simulink model "cmpy3"  (Simulink 6.2)
settings: Solver=ode45  StartTime=0.0  StopTime=10.0  RelTol=1e-3
values from neighbouring files (symbols this model uses):
  h = 50    [fir_init.m]    (also in r2_dit_fft_init.m; r4_dit_fft_init.m = 80)
libraries: xbsIndex_r3 x57
settings Model: LastModifiedBy=mdexter
settings DebuggingCC: SolverPrmCheckMsg=warning

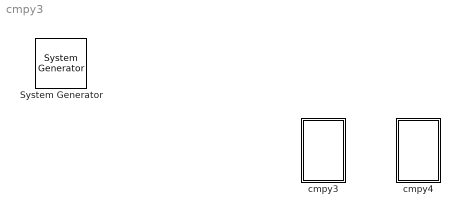
== system cmpy3 ==
  " System Generator" : xbsIndex_r3/ System Generator  Tag=genX  xilinxfamily=Virtex2  part=xc2v1000  speed=-4  package=bg575  synthesis_tool=XST  directory=./netlist  testbench=off  simulink_period=1  sysclk_period=100  incr_netlist=off  trim_vbits=Everywhere in SubSystem  dbl_ovrd=According to Block Masks  core_generation=According to Block Masks  run_coregen=off  deprecated_control=off  eval_field=0
      settings: AttributesFormatString=System\nGenerator
  cmpy3 : Subsystem
  cmpy4 : Subsystem

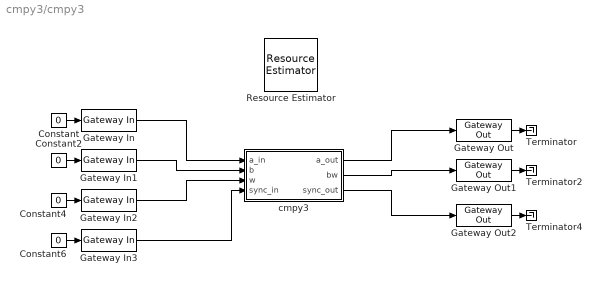
== system cmpy3/cmpy3 ==
  Constant{,2,4,6} (4 alike) : Constant  Value=0
  Gateway In : xbsIndex_r3/Gateway In  arith_type=Unsigned  n_bits=34  bin_pt=0  quantization=Truncate  overflow=Wrap  period=1  timing_constraint=None  locs_specified=off  LOCs={}  needs_fixed_name=off  dbl_ovrd=off  show_param=off
      settings: xl_area=[0 0 0 0 34 0 0]
  Gateway In1 : xbsIndex_r3/Gateway In  arith_type=Unsigned  n_bits=34  bin_pt=0  quantization=Truncate  overflow=Wrap  period=1  timing_constraint=None  locs_specified=off  LOCs={}  needs_fixed_name=off  dbl_ovrd=off  show_param=off
      settings: xl_area=[0 0 0 0 34 0 0]
  Gateway In2 : xbsIndex_r3/Gateway In  arith_type=Unsigned  n_bits=18  bin_pt=0  quantization=Truncate  overflow=Wrap  period=1  timing_constraint=None  locs_specified=off  LOCs={}  needs_fixed_name=off  dbl_ovrd=off  show_param=off
      settings: xl_area=[0 0 0 0 18 0 0]
  Gateway In3 : xbsIndex_r3/Gateway In  arith_type=Boolean  n_bits=8  bin_pt=6  quantization=Truncate  overflow=Wrap  period=1  timing_constraint=None  locs_specified=off  LOCs={}  needs_fixed_name=off  dbl_ovrd=off  show_param=off
      settings: xl_area=[0 0 0 0 1 0 0]
  Gateway Out : xbsIndex_r3/Gateway Out  output_type=Double  nbits=8  bin_pt=6  arith_type=Boolean  quantization=Truncate  overflow=Wrap  hdl_port=on  timing_constraint=None  locs_specified=off  LOCs={}  needs_fixed_name=off  show_param=off
      settings: xl_area=[0 0 0 0 34 0 0]
  Gateway Out1 : xbsIndex_r3/Gateway Out  output_type=Double  nbits=8  bin_pt=6  arith_type=Boolean  quantization=Truncate  overflow=Wrap  hdl_port=on  timing_constraint=None  locs_specified=off  LOCs={}  needs_fixed_name=off  show_param=off
      settings: xl_area=[0 0 0 0 34 0 0]
  Gateway Out2 : xbsIndex_r3/Gateway Out  output_type=Double  nbits=8  bin_pt=6  arith_type=Boolean  quantization=Truncate  overflow=Wrap  hdl_port=on  timing_constraint=None  locs_specified=off  LOCs={}  needs_fixed_name=off  show_param=off
      settings: xl_area=[0 0 0 0 1 0 0]
  Resource Estimator : xbsIndex_r3/Resource Estimator  Tag=resEstTag  xl_estimator_area=[216 323 0 329 156 3 0]  xl_use_estimator_area=off  simulink_period=1  mrp_directory=h:\dev\newfft.fun
      settings: AttributesFormatString=Resource Estimator\n%<xl_estimator_area>\n[SL FF BR LUT IO MUL TBUF]
  Terminator : Terminator
  Terminator2 : Terminator
  Terminator4 : Terminator
  cmpy3 : Subsystem  mask(Complex Multiplier (4 real multipliers)){n_bits_b=8, bin_pt_b=7, n_bits_w=9, bin_pt_w=7, n_bits_bw=8, bin_pt_bw=7, quantization=Round  (unbiased: +/- Inf), overflow=Saturate, mult_latency=3, add_latency=1}
      mask prompts: n_bits_b "Number of Bits B"; bin_pt_b "Binary Point B"; n_bits_w "Number of Bits W"; bin_pt_w "Binary Point W"; n_bits_bw "Number of Bits BW"; bin_pt_bw "Binary Point BW"; mult_latency "Multiplier Latency"; add_latency "Adder Latency"
      mask help: This block multiplies two complex numbers using 4 real multipliers and 2 real adders. Pass-through paths are provided for another complex number and a sync signal. These pass through paths provide delay that matches the latency of the complex multiply operation.
      mask init:
      | cmpy3_init(gcb, ...
      |     n_bits_b,bin_pt_b, ...
      |     n_bits_w,bin_pt_w, ...
      |     n_bits_bw,bin_pt_bw, ...
      |     quantization,overflow, ...
      |     mult_latency,add_latency);
      settings: AttributesFormatString=8_7 * 9_7 ==> 8_7
      mask Help:
      | <pre>
      | Description::
      | 
      | This block multiplies two complex numbers using 4 real multipliers and 2 real adders.
      | Pass-through paths are provided for another complex number and a sync signal.
      | These paths provide delay that matches the latency of the complex multiply operation.
      | 
      | a_in is passed through to a_out.
      | b and w complex inputs are multiplied and their product appears on the bw output.
      | sync_in is passed through to sync_out.
      | 
      | Mask Parameters::
      | 
      | Number of Bits B (n_bits_b): Specifies the width of the real/imaginary
      | components of input b.  Assumed equal for both components.
      | 
      | Binary Point B (bin_pt_b): Specifies the binary point point position of the
      | real/imaginary components of input b.  Assumed equal for both components.
      | 
      | Number of Bits W (n_bits_w): Specifies the width of the real/imaginary
      | components of input w.  Assumed equal for both components.
      | 
      | Binary Point W (bin_pt_w): Specifies the binary point point position of the
      | real/imaginary components of input w.  Assumed equal for both components.
      | 
      | Number of Bits BW (n_bits_bw): Specifies the width of the real/imaginary
      | components of output bw.  Assumed equal for both components.
      | 
      | Binary Point BW (bin_pt_bw): Specifies the binary point point position of the
      | real/imaginary components of output bw.  Assumed equal for both components.
      | 
      | Quantization (quantization): Specifies quantization handling.
      | 
      | Overflow (overflow): Specifies overflow handling.
      | 
      | Multiplier Latency (mult_latency): Latency to use for the underlying real multipliers.
      | 
      | Adder Latency (add_latency): Latency to use for the underlying real adders.
      | </pre>
      mask StyleString: edit,edit,edit,edit,edit,edit,popup(Truncate|Round  (unbiased: +/- Inf)),popup(Wrap|Saturate|Error),edit,edit
  wires:
  Gateway In/1 -> cmpy3/1(a_in)
  cmpy3/1(a_out) -> Gateway Out/1
  Gateway In1/1 -> cmpy3/2(b)
  cmpy3/2(bw) -> Gateway Out1/1
  Gateway In2/1 -> cmpy3/3(w)
  cmpy3/3(sync_out) -> Gateway Out2/1
  Gateway In3/1 -> cmpy3/4(sync_in)
  Constant/1 -> Gateway In/1
  Constant2/1 -> Gateway In1/1
  Constant4/1 -> Gateway In2/1
  Constant6/1 -> Gateway In3/1
  Gateway Out/1 -> Terminator/1
  Gateway Out1/1 -> Terminator2/1
  Gateway Out2/1 -> Terminator4/1

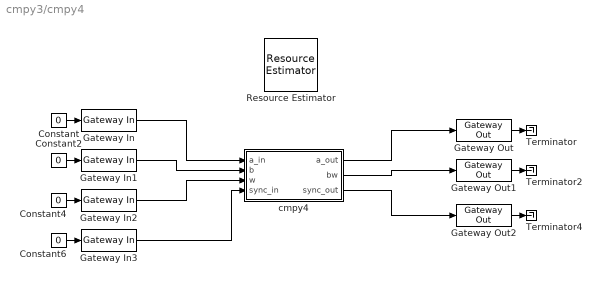
== system cmpy3/cmpy4 ==
  Constant{,2,4,6} (4 alike) : Constant  Value=0
  Gateway In : xbsIndex_r3/Gateway In  arith_type=Unsigned  n_bits=34  bin_pt=0  quantization=Truncate  overflow=Wrap  period=1  timing_constraint=None  locs_specified=off  LOCs={}  needs_fixed_name=off  dbl_ovrd=off  show_param=off
      settings: xl_area=[0 0 0 0 34 0 0]
  Gateway In1 : xbsIndex_r3/Gateway In  arith_type=Unsigned  n_bits=34  bin_pt=0  quantization=Truncate  overflow=Wrap  period=1  timing_constraint=None  locs_specified=off  LOCs={}  needs_fixed_name=off  dbl_ovrd=off  show_param=off
      settings: xl_area=[0 0 0 0 34 0 0]
  Gateway In2 : xbsIndex_r3/Gateway In  arith_type=Unsigned  n_bits=18  bin_pt=0  quantization=Truncate  overflow=Wrap  period=1  timing_constraint=None  locs_specified=off  LOCs={}  needs_fixed_name=off  dbl_ovrd=off  show_param=off
      settings: xl_area=[0 0 0 0 18 0 0]
  Gateway In3 : xbsIndex_r3/Gateway In  arith_type=Boolean  n_bits=8  bin_pt=6  quantization=Truncate  overflow=Wrap  period=1  timing_constraint=None  locs_specified=off  LOCs={}  needs_fixed_name=off  dbl_ovrd=off  show_param=off
      settings: xl_area=[0 0 0 0 1 0 0]
  Gateway Out : xbsIndex_r3/Gateway Out  output_type=Double  nbits=8  bin_pt=6  arith_type=Boolean  quantization=Truncate  overflow=Wrap  hdl_port=on  timing_constraint=None  locs_specified=off  LOCs={}  needs_fixed_name=off  show_param=off
      settings: xl_area=[0 0 0 0 34 0 0]
  Gateway Out1 : xbsIndex_r3/Gateway Out  output_type=Double  nbits=8  bin_pt=6  arith_type=Boolean  quantization=Truncate  overflow=Wrap  hdl_port=on  timing_constraint=None  locs_specified=off  LOCs={}  needs_fixed_name=off  show_param=off
      settings: xl_area=[0 0 0 0 34 0 0]
  Gateway Out2 : xbsIndex_r3/Gateway Out  output_type=Double  nbits=8  bin_pt=6  arith_type=Boolean  quantization=Truncate  overflow=Wrap  hdl_port=on  timing_constraint=None  locs_specified=off  LOCs={}  needs_fixed_name=off  show_param=off
      settings: xl_area=[0 0 0 0 1 0 0]
  Resource Estimator : xbsIndex_r3/Resource Estimator  Tag=resEstTag  xl_estimator_area=[210 297 0 311 156 4 0]  xl_use_estimator_area=off  simulink_period=1  mrp_directory=h:\dev\newfft.fun
      settings: AttributesFormatString=Resource Estimator\n%<xl_estimator_area>\n[SL FF BR LUT IO MUL TBUF]
  Terminator : Terminator
  Terminator2 : Terminator
  Terminator4 : Terminator
  cmpy4 : Subsystem  mask(Complex Multiplier (4 real multipliers)){n_bits_b=17, bin_pt_b=7, n_bits_w=9, bin_pt_w=7, n_bits_bw=17, bin_pt_bw=7, quantization=Round  (unbiased: +/- Inf), overflow=Saturate, mult_latency=3, add_latency=1}
      mask prompts: n_bits_b "Number of Bits B"; bin_pt_b "Binary Point B"; n_bits_w "Number of Bits W"; bin_pt_w "Binary Point W"; n_bits_bw "Number of Bits BW"; bin_pt_bw "Binary Point BW"; mult_latency "Multiplier Latency"; add_latency "Adder Latency"
      mask help: This block multiplies two complex numbers using 4 real multipliers and 2 real adders. Pass-through paths are provided for another complex number and a sync signal. These pass through paths provide delay that matches the latency of the complex multiply operation.
      mask init:
      | cmpy4_init(gcb, ...
      |     n_bits_b,bin_pt_b, ...
      |     n_bits_w,bin_pt_w, ...
      |     n_bits_bw,bin_pt_bw, ...
      |     quantization,overflow, ...
      |     mult_latency,add_latency);
      settings: AttributesFormatString=17_7 * 9_7 ==> 17_7
      mask Help:
      | <pre>
      | Description::
      | 
      | This block multiplies two complex numbers using 4 real multipliers and 2 real adders.
      | Pass-through paths are provided for another complex number and a sync signal.
      | These paths provide delay that matches the latency of the complex multiply operation.
      | 
      | a_in is passed through to a_out.
      | b and w complex inputs are multiplied and their product appears on the bw output.
      | sync_in is passed through to sync_out.
      | 
      | Mask Parameters::
      | 
      | Number of Bits B (n_bits_b): Specifies the width of the real/imaginary
      | components of input b.  Assumed equal for both components.
      | 
      | Binary Point B (bin_pt_b): Specifies the binary point point position of the
      | real/imaginary components of input b.  Assumed equal for both components.
      | 
      | Number of Bits W (n_bits_w): Specifies the width of the real/imaginary
      | components of input w.  Assumed equal for both components.
      | 
      | Binary Point W (bin_pt_w): Specifies the binary point point position of the
      | real/imaginary components of input w.  Assumed equal for both components.
      | 
      | Number of Bits BW (n_bits_bw): Specifies the width of the real/imaginary
      | components of output bw.  Assumed equal for both components.
      | 
      | Binary Point BW (bin_pt_bw): Specifies the binary point point position of the
      | real/imaginary components of output bw.  Assumed equal for both components.
      | 
      | Quantization (quantization): Specifies quantization handling.
      | 
      | Overflow (overflow): Specifies overflow handling.
      | 
      | Multiplier Latency (mult_latency): Latency to use for the underlying real multipliers.
      | 
      | Adder Latency (add_latency): Latency to use for the underlying real adders.
      | </pre>
      mask StyleString: edit,edit,edit,edit,edit,edit,popup(Truncate|Round  (unbiased: +/- Inf)),popup(Wrap|Saturate|Error),edit,edit
  wires:
  Gateway In/1 -> cmpy4/1(a_in)
  cmpy4/1(a_out) -> Gateway Out/1
  Gateway In1/1 -> cmpy4/2(b)
  cmpy4/2(bw) -> Gateway Out1/1
  Gateway In2/1 -> cmpy4/3(w)
  cmpy4/3(sync_out) -> Gateway Out2/1
  Gateway In3/1 -> cmpy4/4(sync_in)
  Constant/1 -> Gateway In/1
  Constant2/1 -> Gateway In1/1
  Constant4/1 -> Gateway In2/1
  Constant6/1 -> Gateway In3/1
  Gateway Out/1 -> Terminator/1
  Gateway Out1/1 -> Terminator2/1
  Gateway Out2/1 -> Terminator4/1

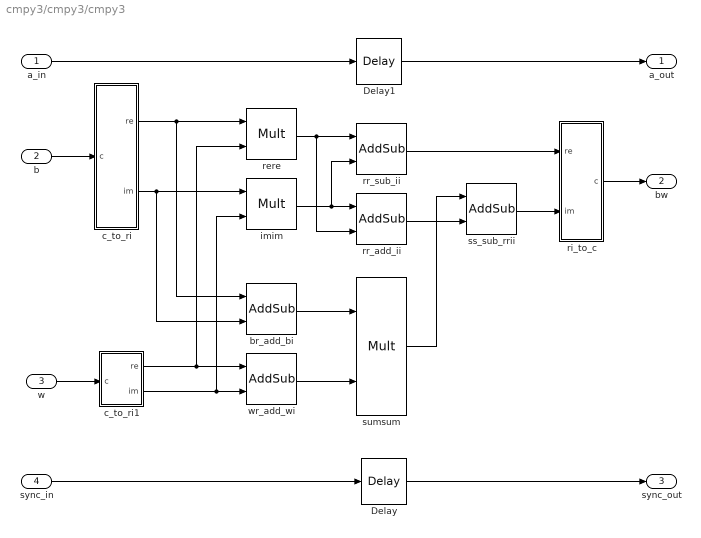
== system cmpy3/cmpy3/cmpy3 ==
  a_in : Inport  Port=1  LatchInput=off
  b : Inport  Port=2  LatchInput=off
  w : Inport  Port=3  LatchInput=off
  sync_in : Inport  Port=4  LatchInput=off
  Delay : xbsIndex_r3/Delay  latency=5  reg_retiming=off  explicit_period=off  period=1  en=off  accept_only_valid=off  init_zero=on  dbl_ovrd=off  show_param=off
      settings: xl_area=[1 1 0 1 0 0 0]
  Delay1 : xbsIndex_r3/Delay  latency=5  reg_retiming=off  explicit_period=off  period=1  en=off  accept_only_valid=off  init_zero=on  dbl_ovrd=off  show_param=off
      settings: xl_area=[17 34 0 34 0 0 0]
  br_add_bi : xbsIndex_r3/AddSub  mode=Addition  precision=Full  arith_type=Unsigned  n_bits=8  bin_pt=2  quantization=Truncate  overflow=Wrap  latency=1  explicit_period=off  period=1  use_carryin=off  use_carryout=off  en=off  dbl_ovrd=off  show_param=on  use_core=on  pipeline=on  use_rpm=on  gen_core=off
      settings: xl_area=[9 18 0 18 0 0 0]
  c_to_ri : Subsystem  mask(Complex to Real-Imag){n_bits=8, bin_pt=7}
      mask prompts: n_bits "Bit Width"; bin_pt "Binary Point"
      mask help: Outputs real and imaginary components of a complex input.
      settings: AttributesFormatString=8_7 r/i
      mask Help:
      | <pre>
      | Description::
      | 
      | Outputs real and imaginary components of a complex input.
      | Useful for simplifying interconnects.
      | See also: Real-Imag to Complex (ri_to_c)
      | 
      | Mask Parameters::
      | 
      | Bit Width (n_bits): Specifies the width of the real/imaginary components.
      | Assumed equal for both components.
      | 
      | Binary Point (bin_pt): Specifies the binary point location in the real/imaginary components.
      | Assumed equal for both components.
      | </pre>
  c_to_ri1 : Subsystem  mask(Complex to Real-Imag){n_bits=9, bin_pt=7}
      mask prompts: n_bits "Bit Width"; bin_pt "Binary Point"
      mask help: Outputs real and imaginary components of a complex input.
      mask init:
      | c_to_ri_init(gcb,n_bits,bin_pt);
      settings: AttributesFormatString=9_7 r/i
      mask Help:
      | <pre>
      | Description::
      | 
      | Outputs real and imaginary components of a complex input.
      | Useful for simplifying interconnects.
      | See also: Real-Imag to Complex (ri_to_c)
      | 
      | Mask Parameters::
      | 
      | Bit Width (n_bits): Specifies the width of the real/imaginary components.
      | Assumed equal for both components.
      | 
      | Binary Point (bin_pt): Specifies the binary point location in the real/imaginary components.
      | Assumed equal for both components.
      | </pre>
  imim : xbsIndex_r3/Mult  precision=Full  arith_type="Signed  (2's comp)"  n_bits=8  bin_pt=2  quantization=Truncate  overflow=Wrap  latency=3  explicit_period=off  period=1  en=off  dbl_ovrd=off  show_param=on  mult_type=Parallel  oversample=2  use_embedded=on  pipeline=on  use_rpm=on  placement_style=Rectangular Shape  gen_core=off
      settings: xl_area=[26 52 0 26 0 1 0]
  rere : xbsIndex_r3/Mult  precision=Full  arith_type="Signed  (2's comp)"  n_bits=8  bin_pt=2  quantization=Truncate  overflow=Wrap  latency=3  explicit_period=off  period=1  en=off  dbl_ovrd=off  show_param=on  mult_type=Parallel  oversample=2  use_embedded=on  pipeline=on  use_rpm=on  placement_style=Rectangular Shape  gen_core=off
      settings: xl_area=[26 52 0 26 0 1 0]
  ri_to_c : Subsystem  mask(Real-Imag to Complex){}
      mask help: Concatenates real and imaginary inputs into a complex output.
      mask init:
      | ri_to_c_init(gcb);
      mask Help:
      | <pre>
      | Description::
      | 
      | Concatenates a real and imaginary input into a complex output.
      | Useful for simplifying interconnects.
      | See also: Complex to Real-Imag (c_to_ri)
      | 
      | Mask Parameters::
      | 
      | (N/A)
      | </pre>
  rr_add_ii : xbsIndex_r3/AddSub  mode=Addition  precision=Full  arith_type=Unsigned  n_bits=8  bin_pt=2  quantization=Truncate  overflow=Wrap  latency=1  explicit_period=off  period=1  use_carryin=off  use_carryout=off  en=off  dbl_ovrd=off  show_param=on  use_core=on  pipeline=on  use_rpm=on  gen_core=off
      settings: xl_area=[14 27 0 27 0 0 0]
  rr_sub_ii : xbsIndex_r3/AddSub  mode=Subtraction  precision=User Defined  arith_type=Unsigned  n_bits=8  bin_pt=7  quantization="Round  (unbiased: +/- Inf)"  overflow=Saturate  latency=2  explicit_period=off  period=1  use_carryin=off  use_carryout=off  en=off  dbl_ovrd=off  show_param=on  use_core=on  pipeline=on  use_rpm=on  gen_core=off
      settings: xl_area=[44 44 0 69 0 0 0]
  ss_sub_rrii : xbsIndex_r3/AddSub  mode=Subtraction  precision=User Defined  arith_type="Signed  (2's comp)"  n_bits=8  bin_pt=7  quantization="Round  (unbiased: +/- Inf)"  overflow=Saturate  latency=1  explicit_period=off  period=1  use_carryin=off  use_carryout=off  en=off  dbl_ovrd=off  show_param=on  use_core=on  pipeline=on  use_rpm=on  gen_core=off
      settings: xl_area=[46 29 0 90 0 0 0]
  sumsum : xbsIndex_r3/Mult  precision=Full  arith_type="Signed  (2's comp)"  n_bits=8  bin_pt=2  quantization=Truncate  overflow=Wrap  latency=3  explicit_period=off  period=1  en=off  dbl_ovrd=off  show_param=on  mult_type=Parallel  oversample=2  use_embedded=on  pipeline=on  use_rpm=on  placement_style=Rectangular Shape  gen_core=off
      settings: xl_area=[28 56 0 28 0 1 0]
  wr_add_wi : xbsIndex_r3/AddSub  mode=Addition  precision=Full  arith_type=Unsigned  n_bits=8  bin_pt=2  quantization=Truncate  overflow=Wrap  latency=1  explicit_period=off  period=1  use_carryin=off  use_carryout=off  en=off  dbl_ovrd=off  show_param=on  use_core=on  pipeline=on  use_rpm=on  gen_core=off
      settings: xl_area=[5 10 0 10 0 0 0]
  a_out : Outport
  bw : Outport  Port=2
  sync_out : Outport  Port=3
  wires:
  Delay1/1 -> a_out/1
  a_in/1 -> Delay1/1
  c_to_ri/2(im) -> imim/1, br_add_bi/2
  c_to_ri1/1(re) -> wr_add_wi/1, rere/2
  c_to_ri1/2(im) -> wr_add_wi/2, imim/2
  c_to_ri/1(re) -> rere/1, br_add_bi/1
  Delay/1 -> sync_out/1
  sync_in/1 -> Delay/1
  sumsum/1 -> ss_sub_rrii/1
  ri_to_c/1(c) -> bw/1
  wr_add_wi/1 -> sumsum/2
  br_add_bi/1 -> sumsum/1
  imim/1 -> rr_add_ii/1, rr_sub_ii/2
  rere/1 -> rr_sub_ii/1, rr_add_ii/2
  w/1 -> c_to_ri1/1(c)
  b/1 -> c_to_ri/1(c)
  rr_add_ii/1 -> ss_sub_rrii/2
  rr_sub_ii/1 -> ri_to_c/1(re)
  ss_sub_rrii/1 -> ri_to_c/2(im)

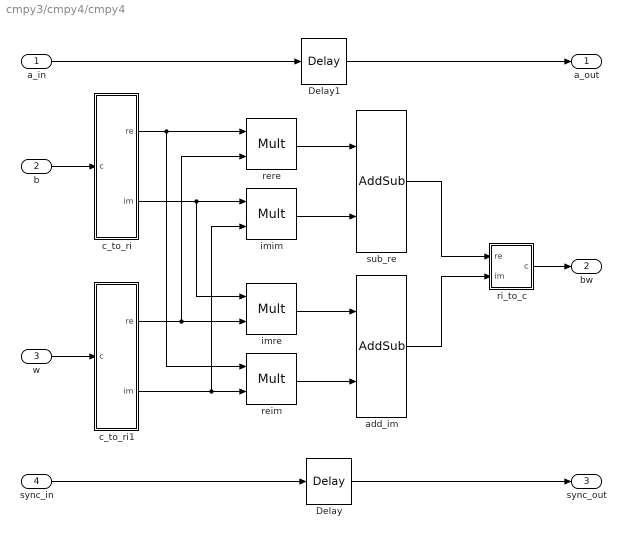
== system cmpy3/cmpy4/cmpy4 ==
  a_in : Inport  Port=1  LatchInput=off
  b : Inport  Port=2  LatchInput=off
  w : Inport  Port=3  LatchInput=off
  sync_in : Inport  Port=4  LatchInput=off
  Delay : xbsIndex_r3/Delay  latency=4  reg_retiming=off  explicit_period=off  period=1  en=off  accept_only_valid=off  init_zero=on  dbl_ovrd=off  show_param=off
      settings: xl_area=[1 1 0 1 0 0 0]
  Delay1 : xbsIndex_r3/Delay  latency=4  reg_retiming=off  explicit_period=off  period=1  en=off  accept_only_valid=off  init_zero=on  dbl_ovrd=off  show_param=off
      settings: xl_area=[17 34 0 34 0 0 0]
  add_im : xbsIndex_r3/AddSub  mode=Addition  precision=User Defined  arith_type="Signed  (2's comp)"  n_bits=17  bin_pt=7  quantization="Round  (unbiased: +/- Inf)"  overflow=Saturate  latency=1  explicit_period=off  period=1  use_carryin=off  use_carryout=off  en=off  dbl_ovrd=off  show_param=on  use_core=on  pipeline=on  use_rpm=on  gen_core=off
      settings: xl_area=[44 27 0 86 0 0 0]
  c_to_ri : Subsystem  mask(Complex to Real-Imag){n_bits=17, bin_pt=7}
      mask prompts: n_bits "Bit Width"; bin_pt "Binary Point"
      mask help: Outputs real and imaginary components of a complex input.
      settings: AttributesFormatString=17_7 r/i
      mask Help:
      | <pre>
      | Description::
      | 
      | Outputs real and imaginary components of a complex input.
      | Useful for simplifying interconnects.
      | See also: Real-Imag to Complex (ri_to_c)
      | 
      | Mask Parameters::
      | 
      | Bit Width (n_bits): Specifies the width of the real/imaginary components.
      | Assumed equal for both components.
      | 
      | Binary Point (bin_pt): Specifies the binary point location in the real/imaginary components.
      | Assumed equal for both components.
      | </pre>
  c_to_ri1 : Subsystem  mask(Complex to Real-Imag){n_bits=9, bin_pt=7}
      mask prompts: n_bits "Bit Width"; bin_pt "Binary Point"
      mask help: Outputs real and imaginary components of a complex input.
      settings: AttributesFormatString=9_7 r/i
      mask Help:
      | <pre>
      | Description::
      | 
      | Outputs real and imaginary components of a complex input.
      | Useful for simplifying interconnects.
      | See also: Real-Imag to Complex (ri_to_c)
      | 
      | Mask Parameters::
      | 
      | Bit Width (n_bits): Specifies the width of the real/imaginary components.
      | Assumed equal for both components.
      | 
      | Binary Point (bin_pt): Specifies the binary point location in the real/imaginary components.
      | Assumed equal for both components.
      | </pre>
  imim : xbsIndex_r3/Mult  precision=Full  arith_type="Signed  (2's comp)"  n_bits=8  bin_pt=2  quantization=Truncate  overflow=Wrap  latency=3  explicit_period=off  period=1  en=off  dbl_ovrd=off  show_param=on  mult_type=Parallel  oversample=2  use_embedded=on  pipeline=on  use_rpm=on  placement_style=Rectangular Shape  gen_core=off
      settings: xl_area=[26 52 0 26 0 1 0]
  imre : xbsIndex_r3/Mult  precision=Full  arith_type="Signed  (2's comp)"  n_bits=8  bin_pt=2  quantization=Truncate  overflow=Wrap  latency=3  explicit_period=off  period=1  en=off  dbl_ovrd=off  show_param=on  mult_type=Parallel  oversample=2  use_embedded=on  pipeline=on  use_rpm=on  placement_style=Rectangular Shape  gen_core=off
      settings: xl_area=[26 52 0 26 0 1 0]
  reim : xbsIndex_r3/Mult  precision=Full  arith_type="Signed  (2's comp)"  n_bits=8  bin_pt=2  quantization=Truncate  overflow=Wrap  latency=3  explicit_period=off  period=1  en=off  dbl_ovrd=off  show_param=on  mult_type=Parallel  oversample=2  use_embedded=on  pipeline=on  use_rpm=on  placement_style=Rectangular Shape  gen_core=off
      settings: xl_area=[26 52 0 26 0 1 0]
  rere : xbsIndex_r3/Mult  precision=Full  arith_type="Signed  (2's comp)"  n_bits=8  bin_pt=2  quantization=Truncate  overflow=Wrap  latency=3  explicit_period=off  period=1  en=off  dbl_ovrd=off  show_param=on  mult_type=Parallel  oversample=2  use_embedded=on  pipeline=on  use_rpm=on  placement_style=Rectangular Shape  gen_core=off
      settings: xl_area=[26 52 0 26 0 1 0]
  ri_to_c : Subsystem  mask(Real-Imag to Complex){}
      mask help: Concatenates real and imaginary inputs into a complex output.
      mask init:
      | ri_to_c_init(gcb);
      mask Help:
      | <pre>
      | Description::
      | 
      | Concatenates a real and imaginary input into a complex output.
      | Useful for simplifying interconnects.
      | See also: Complex to Real-Imag (c_to_ri)
      | 
      | Mask Parameters::
      | 
      | (N/A)
      | </pre>
  sub_re : xbsIndex_r3/AddSub  mode=Subtraction  precision=User Defined  arith_type="Signed  (2's comp)"  n_bits=17  bin_pt=7  quantization="Round  (unbiased: +/- Inf)"  overflow=Saturate  latency=1  explicit_period=off  period=1  use_carryin=off  use_carryout=off  en=off  dbl_ovrd=off  show_param=on  use_core=on  pipeline=on  use_rpm=on  gen_core=off
      settings: xl_area=[44 27 0 86 0 0 0]
  a_out : Outport
  bw : Outport  Port=2
  sync_out : Outport  Port=3
  wires:
  Delay1/1 -> a_out/1
  a_in/1 -> Delay1/1
  c_to_ri/2(im) -> imre/1, imim/1
  c_to_ri1/1(re) -> rere/2, imre/2
  c_to_ri1/2(im) -> imim/2, reim/2
  c_to_ri/1(re) -> reim/1, rere/1
  Delay/1 -> sync_out/1
  sync_in/1 -> Delay/1
  add_im/1 -> ri_to_c/2(im)
  ri_to_c/1(c) -> bw/1
  sub_re/1 -> ri_to_c/1(re)
  reim/1 -> add_im/2
  imre/1 -> add_im/1
  imim/1 -> sub_re/2
  rere/1 -> sub_re/1
  w/1 -> c_to_ri1/1(c)
  b/1 -> c_to_ri/1(c)

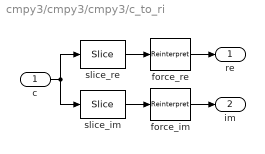
== system cmpy3/cmpy3/cmpy3/c_to_ri ==
  c : Inport  Port=1  LatchInput=off
  force_im : xbsIndex_r3/Reinterpret  force_arith_type=on  arith_type="Signed  (2's comp)"  force_bin_pt=on  bin_pt=7  force_valid=on
  force_re : xbsIndex_r3/Reinterpret  force_arith_type=on  arith_type="Signed  (2's comp)"  force_bin_pt=on  bin_pt=7  force_valid=on
  slice_im : xbsIndex_r3/Slice  mode=Lower Bit Location + Width  nbits=8  bit1=0  base1=MSB of Input  bit0=0  base0=LSB of Input  boolean_output=off  explicit_period=off  period=1  dbl_ovrd=off
  slice_re : xbsIndex_r3/Slice  mode=Upper Bit Location + Width  nbits=8  bit1=0  base1=MSB of Input  bit0=0  base0=LSB of Input  boolean_output=off  explicit_period=off  period=1  dbl_ovrd=off
  re : Outport
  im : Outport  Port=2
  wires:
  slice_re/1 -> force_re/1
  slice_im/1 -> force_im/1
  force_re/1 -> re/1
  force_im/1 -> im/1
  c/1 -> slice_re/1, slice_im/1

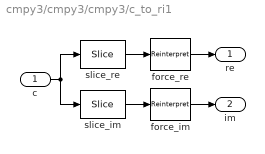
== system cmpy3/cmpy3/cmpy3/c_to_ri1 ==
  c : Inport  Port=1  LatchInput=off
  force_im : xbsIndex_r3/Reinterpret  force_arith_type=on  arith_type="Signed  (2's comp)"  force_bin_pt=on  bin_pt=7  force_valid=on
  force_re : xbsIndex_r3/Reinterpret  force_arith_type=on  arith_type="Signed  (2's comp)"  force_bin_pt=on  bin_pt=7  force_valid=on
  slice_im : xbsIndex_r3/Slice  mode=Lower Bit Location + Width  nbits=9  bit1=0  base1=MSB of Input  bit0=0  base0=LSB of Input  boolean_output=off  explicit_period=off  period=1  dbl_ovrd=off
  slice_re : xbsIndex_r3/Slice  mode=Upper Bit Location + Width  nbits=9  bit1=0  base1=MSB of Input  bit0=0  base0=LSB of Input  boolean_output=off  explicit_period=off  period=1  dbl_ovrd=off
  re : Outport
  im : Outport  Port=2
  wires:
  c/1 -> slice_im/1, slice_re/1
  force_im/1 -> im/1
  force_re/1 -> re/1
  slice_im/1 -> force_im/1
  slice_re/1 -> force_re/1

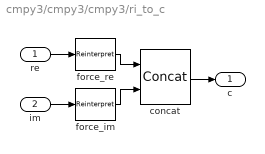
== system cmpy3/cmpy3/cmpy3/ri_to_c ==
  re : Inport  Port=1  LatchInput=off
  im : Inport  Port=2  LatchInput=off
  concat : xbsIndex_r3/Concat  num_inputs=2  explicit_period=off  period=1  dbl_ovrd=off
  force_im : xbsIndex_r3/Reinterpret  force_arith_type=on  arith_type=Unsigned  force_bin_pt=on  bin_pt=0  force_valid=on
  force_re : xbsIndex_r3/Reinterpret  force_arith_type=on  arith_type=Unsigned  force_bin_pt=on  bin_pt=0  force_valid=on
  c : Outport
  wires:
  im/1 -> force_im/1
  concat/1 -> c/1
  re/1 -> force_re/1
  force_im/1 -> concat/2
  force_re/1 -> concat/1

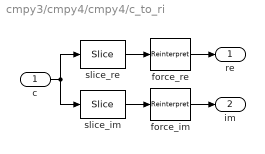
== system cmpy3/cmpy4/cmpy4/c_to_ri ==
  c : Inport  Port=1  LatchInput=off
  force_im : xbsIndex_r3/Reinterpret  force_arith_type=on  arith_type="Signed  (2's comp)"  force_bin_pt=on  bin_pt=7  force_valid=on
  force_re : xbsIndex_r3/Reinterpret  force_arith_type=on  arith_type="Signed  (2's comp)"  force_bin_pt=on  bin_pt=7  force_valid=on
  slice_im : xbsIndex_r3/Slice  mode=Lower Bit Location + Width  nbits=17  bit1=0  base1=MSB of Input  bit0=0  base0=LSB of Input  boolean_output=off  explicit_period=off  period=1  dbl_ovrd=off
  slice_re : xbsIndex_r3/Slice  mode=Upper Bit Location + Width  nbits=17  bit1=0  base1=MSB of Input  bit0=0  base0=LSB of Input  boolean_output=off  explicit_period=off  period=1  dbl_ovrd=off
  re : Outport
  im : Outport  Port=2
  wires:
  slice_re/1 -> force_re/1
  slice_im/1 -> force_im/1
  force_re/1 -> re/1
  force_im/1 -> im/1
  c/1 -> slice_re/1, slice_im/1

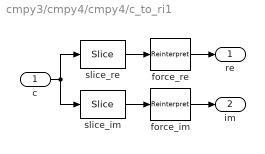
== system cmpy3/cmpy4/cmpy4/c_to_ri1 ==
  c : Inport  Port=1  LatchInput=off
  force_im : xbsIndex_r3/Reinterpret  force_arith_type=on  arith_type="Signed  (2's comp)"  force_bin_pt=on  bin_pt=7  force_valid=on
  force_re : xbsIndex_r3/Reinterpret  force_arith_type=on  arith_type="Signed  (2's comp)"  force_bin_pt=on  bin_pt=7  force_valid=on
  slice_im : xbsIndex_r3/Slice  mode=Lower Bit Location + Width  nbits=9  bit1=0  base1=MSB of Input  bit0=0  base0=LSB of Input  boolean_output=off  explicit_period=off  period=1  dbl_ovrd=off
  slice_re : xbsIndex_r3/Slice  mode=Upper Bit Location + Width  nbits=9  bit1=0  base1=MSB of Input  bit0=0  base0=LSB of Input  boolean_output=off  explicit_period=off  period=1  dbl_ovrd=off
  re : Outport
  im : Outport  Port=2
  wires:
  slice_re/1 -> force_re/1
  slice_im/1 -> force_im/1
  force_re/1 -> re/1
  force_im/1 -> im/1
  c/1 -> slice_re/1, slice_im/1

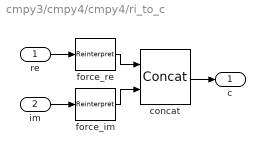
== system cmpy3/cmpy4/cmpy4/ri_to_c ==
  re : Inport  Port=1  LatchInput=off
  im : Inport  Port=2  LatchInput=off
  concat : xbsIndex_r3/Concat  num_inputs=2  explicit_period=off  period=1  dbl_ovrd=off
  force_im : xbsIndex_r3/Reinterpret  force_arith_type=on  arith_type=Unsigned  force_bin_pt=on  bin_pt=0  force_valid=on
  force_re : xbsIndex_r3/Reinterpret  force_arith_type=on  arith_type=Unsigned  force_bin_pt=on  bin_pt=0  force_valid=on
  c : Outport
  wires:
  im/1 -> force_im/1
  concat/1 -> c/1
  re/1 -> force_re/1
  force_im/1 -> concat/2
  force_re/1 -> concat/1
